simulink model "homework_4_2"  (R2023a)
settings: Solver=VariableStepAuto  StartTime=0.0  StopTime=2  MaxStep=Te / 10  RelTol=1e-6
undefined symbols (not defined in the file): beta, Ce, Cm, R, Te, Tm
settings Model: Creator=matve  LastModifiedBy=matve

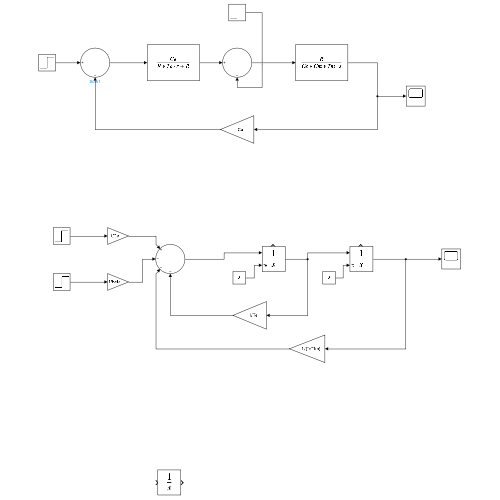
[thumbnail: Simulink's stored preview of the top-level diagram]
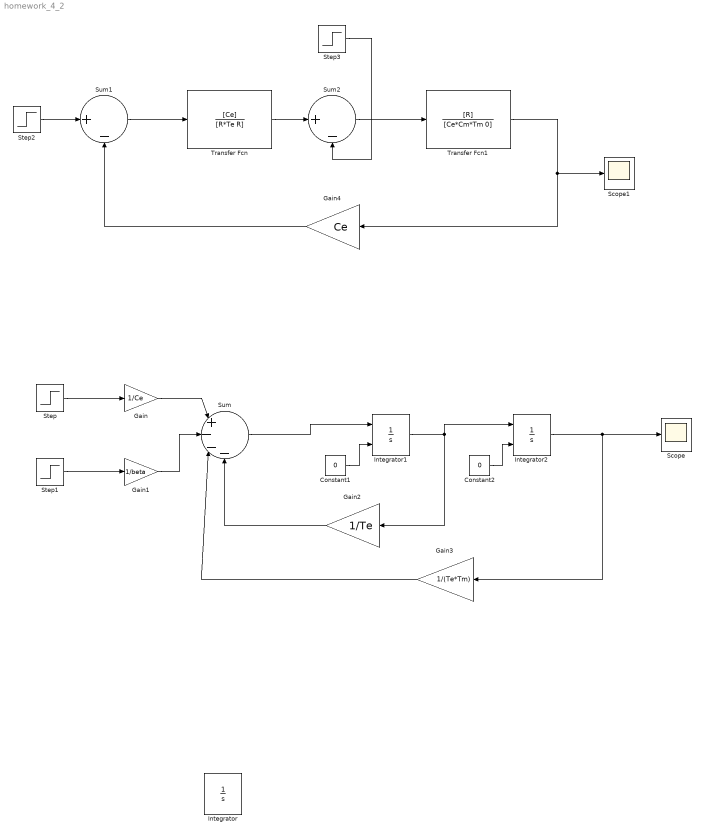
== system homework_4_2 ==
  Constant1 : Constant  Value=0
  Constant2 : Constant  Value=0
  Gain : Gain  Gain=1/Ce
  Gain1 : Gain  Gain=1/beta
  Gain2 : Gain  Gain=1/Te
  Gain3 : Gain  Gain=1/(Te*Tm)
  Gain4 : Gain  Gain=Ce
  Integrator : Integrator
  Integrator1 : Integrator  InitialConditionSource=external  ShowStatePort=on
  Integrator2 : Integrator  InitialConditionSource=external  ShowStatePort=on
  Scope : Scope
  Scope1 : Scope
  Step : Step  Time=0  After=270  SampleTime=0
  Step1 : Step  Time=10*Tm  After=2.046  SampleTime=0
  Step2 : Step  Time=0  After=270  SampleTime=0
  Step3 : Step  Time=10*Tm  After=2.046  SampleTime=0
  Sum : Sum  Inputs=|+---
  Sum1 : Sum  Inputs=|+-
  Sum2 : Sum  Inputs=|+-
  Transfer Fcn : TransferFcn  Numerator=[Ce]  Denominator=[R*Te R]
  Transfer Fcn1 : TransferFcn  Numerator=[R]  Denominator=[Ce*Cm*Tm 0]
  wires:
  Step/1 -> Gain/1
  Step1/1 -> Gain1/1
  Gain/1 -> Sum/1
  Gain1/1 -> Sum/2
  Sum/1 -> Integrator1/1
  Integrator1/1 -> Integrator2/1, Gain2/1
  Gain2/1 -> Sum/4
  Integrator2/1 -> Gain3/1, Scope/1
  Gain3/1 -> Sum/3
  Constant1/1 -> Integrator1/2
  Constant2/1 -> Integrator2/2
  Step2/1 -> Sum1/1
  Sum1/1 -> Transfer Fcn/1
  Transfer Fcn/1 -> Sum2/1
  Sum2/1 -> Transfer Fcn1/1
  Transfer Fcn1/1 -> Gain4/1, Scope1/1
  Gain4/1 -> Sum1/2
  Step3/1 -> Sum2/2
